simulink model "feedbackPID"  (Simulink 6.1)
settings: Solver=ode45  StartTime=0.0  StopTime=20.0  RelTol=1e-3
settings Model: LastModifiedBy=okawa
settings DebuggingCC: SolverPrmCheckMsg=warning

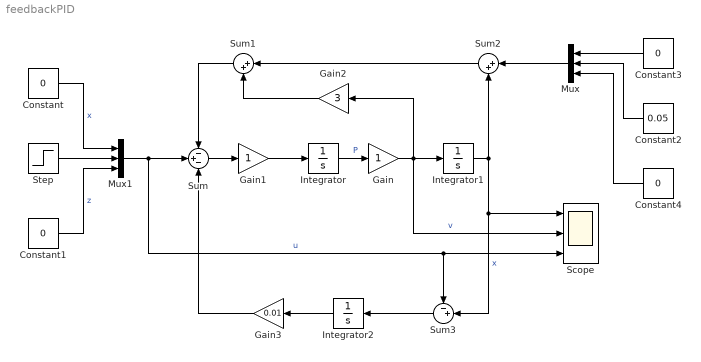
== system feedbackPID ==
  Constant : Constant  Value=0
  Constant1 : Constant  Value=0
  Constant2 : Constant  Orientation=left  Value=0.05
  Constant3 : Constant  Orientation=left  Value=0
  Constant4 : Constant  Orientation=left  Value=0
  Gain : Gain
  Gain1 : Gain
  Gain2 : Gain  Orientation=left  Gain=3
  Gain3 : Gain  Orientation=left  Gain=0.01
  Integrator : Integrator
  Integrator1 : Integrator
  Integrator2 : Integrator  Orientation=left
  Mux : Mux  Orientation=left  Inputs=3
  Mux1 : Mux  Inputs=3
  Scope : Scope  NumInputPorts=3
      settings: YMin=-5~-5~-5  YMax=5~5~5
  Step : Step  SampleTime=0
  Sum : Sum  Inputs=-+-
  Sum1 : Sum  Orientation=left  Inputs=|++
  Sum2 : Sum  Orientation=left  Inputs=|++
  Sum3 : Sum  Orientation=left  Inputs=-+|
  wires:
  Constant/1 -> Mux1/1  "x"
  Constant1/1 -> Mux1/3  "z"
  Integrator1/1 -> Sum2/2, Scope/1, Sum3/2  "x"
  Integrator/1 -> Gain/1  "P"
  Gain/1 -> Integrator1/1, Scope/2, Gain2/1  "v"
  Mux1/1 -> Sum/2, Scope/3, Sum3/1  "u"
  Step/1 -> Mux1/2
  Sum/1 -> Gain1/1
  Gain1/1 -> Integrator/1
  Sum1/1 -> Sum/1
  Gain2/1 -> Sum1/2
  Sum2/1 -> Sum1/1
  Constant3/1 -> Mux/1
  Constant2/1 -> Mux/2
  Constant4/1 -> Mux/3
  Mux/1 -> Sum2/1
  Integrator2/1 -> Gain3/1
  Gain3/1 -> Sum/3
  Sum3/1 -> Integrator2/1
